simulink model "drone_PID"  (R2021a)
settings: Solver=FixedStepAuto  StartTime=0.0  StopTime=10.0  RelTol=1e-3  EnableMultiTasking=on
model workspace (MAT data in the model file):
  Ts = 0.016
undefined symbols (not defined in the file or in its folder): AUX, dev, DiscIntNeverNeededParam, pwm_output1
libraries: px4Sensorslib x8, px4lib x4, cstblocks x3, simulink x1
settings Model: ExtModeTrigDuration=10  Creator=Kawaguchi  LastModifiedBy=beket
settings SolverCC: PositivePriorityOrder=on
settings OptimizationCC: EnhancedBackFolding=on  PassReuseOutputArgsAs=Individual arguments  ZeroExternalMemoryAtStartup=off  ZeroInternalMemoryAtStartup=off  MaxStackSize=64  OptimizeBlockOrder=speed  DifferentSizesBufferReuse=on  OptimizationCustomize=off  EfficientTunableParamExpr=on
settings DebuggingCC: ParameterTunabilityLossMsg=error
settings HardwareCC: ProdBitPerPointer=32  ProdBitPerSizeT=32  ProdBitPerPtrDiffT=32  ProdLargestAtomicInteger=Long  ProdLargestAtomicFloat=Double  ProdWordSize=32  ProdLongLongMode=on  ProdHWDeviceType=ARM Compatible->ARM Cortex
settings SFSimCC: MATLABDynamicMemAlloc=off  SimTargetLang=C++
settings RTWCC: SystemTargetFile=ert.tlc  HardwareBoard=PX4 Pixhawk 4  TLCOptions="-aInlineSetEventsForThisBaseRateFcn=TLC_FALSE -aSuppressMultiTaskScheduler=TLC_FALSE  -aRateBasedStepFcn=0"  TemplateMakefile=ert_default_tmf  Toolchain=GNU Tools for PX4 Autopilots  TargetLang=C++
settings CodeAppCC: ForceParamTrailComments=on  IgnoreCustomStorageClasses=off  OperatorAnnotations=on  SimulinkDataObjDesc=on  SFDataObjDesc=on  InsertBlockDesc=on
settings ERTTargetCC: ExtModeTransport=3  ExtModeStaticAlloc=on  ExtModeStaticAllocSize=1024  ExtModeMexFile=ext_xcp  ExtModeIntrfLevel=Level2 - Open

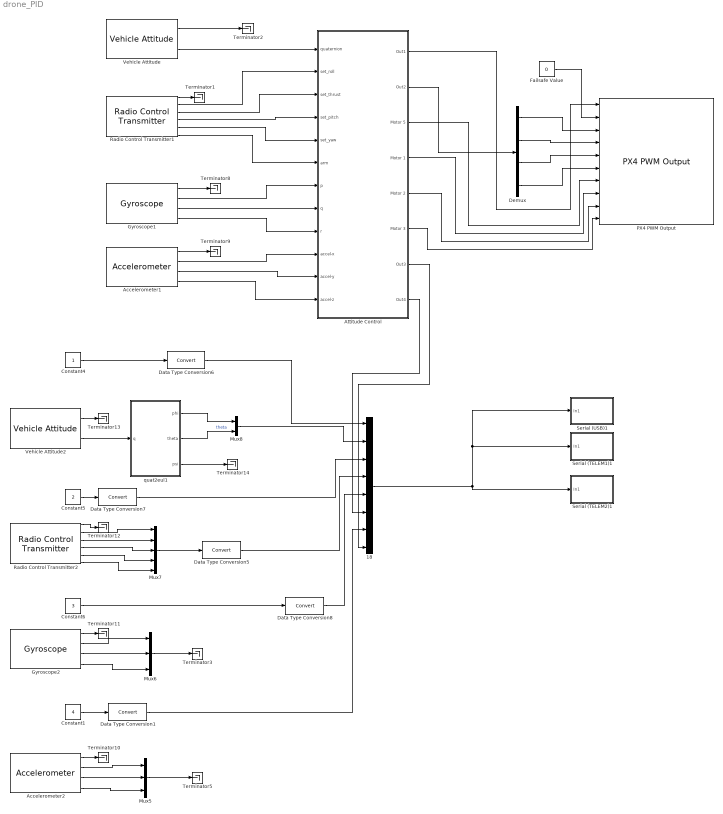
== system drone_PID ==
  18 : Mux  Inputs=8
  Accelerometer1 : px4Sensorslib/Accelerometer  uorbTimeStamp=off  BlockingMode=off  BlockTimeout=1e-3  sampleTime=1/250
      settings: SourceProductBaseCode=PX4AUTOPILOTS
  Accelerometer2 : px4Sensorslib/Accelerometer  uorbTimeStamp=off  BlockingMode=off  BlockTimeout=1e-3  sampleTime=Ts
      settings: SourceProductBaseCode=PX4AUTOPILOTS
  Attitude Control : Subsystem
  Constant1 : Constant  Value=4
  Constant4 : Constant
  Constant5 : Constant  Value=2
  Constant6 : Constant  Value=3
  Data Type Conversion{1,5..8} (5 alike) : DataTypeConversion
  Demux : Demux
  Failsafe Value : Constant  Value=0  OutDataTypeStr=boolean  SampleTime=-1
  Gyroscope1 : px4Sensorslib/Gyroscope  uorbTimeStamp=off  BlockingMode=off  BlockTimeout=1e-3  sampleTime=1/250
      settings: SourceProductBaseCode=PX4AUTOPILOTS
  Gyroscope2 : px4Sensorslib/Gyroscope  uorbTimeStamp=off  BlockingMode=off  BlockTimeout=1e-3  sampleTime=Ts
      settings: SourceProductBaseCode=PX4AUTOPILOTS
  Mux5 : Mux  Inputs=3
  Mux6 : Mux  Inputs=3
  Mux7 : Mux  Inputs=5
  Mux8 : Mux  Inputs=2
  PX4 PWM Output : px4lib/PX4 PWM Output  pwmDevice=AUX (/dev/pwm_output1)  pwmChannel1_=on  pwmChannel2_=on  pwmChannel3_=on  pwmChannel4_=on  pwmChannel5_=on  pwmChannel6_=on  pwmChannel7_=on  pwmChannel8_=on  forceTerminateFailsafe=off  outputErrorStatus=off
      settings: SourceProductBaseCode=PX4AUTOPILOTS
  Radio Control Transmitter1 : px4Sensorslib/Radio Control Transmitter  channel1=on  channel2=on  channel3=on  channel4=on  channel5=on  channel6=off  channel7=off  channel8=off  channel_count=off  rssi=off  rc_input_source=off  timestamp_last_signal=off  time_stamp=off  sampleTime=1/250  BlockingMode=off  BlockTimeout=5
      settings: SourceProductBaseCode=PX4AUTOPILOTS
  Radio Control Transmitter2 : px4Sensorslib/Radio Control Transmitter  channel1=on  channel2=on  channel3=on  channel4=on  channel5=on  channel6=off  channel7=off  channel8=off  channel_count=off  rssi=off  rc_input_source=off  timestamp_last_signal=off  time_stamp=off  sampleTime=Ts  BlockingMode=off  BlockTimeout=5
      settings: SourceProductBaseCode=PX4AUTOPILOTS
  Serial (TELEM1)1 : Subsystem
  Serial (TELEM2)1 : Subsystem
  Serial (USB)1 : Subsystem
  Terminator{1..3,5,8..14} (11 alike) : Terminator
  Vehicle Attitude : px4Sensorslib/Vehicle Attitude  rollRate=off  pitchRate=off  yawRate=off  quaternion=on  uorbTimeStamp=off  BlockingMode=off  BlockTimeout=0.001  sampleTime=1/250
      settings: SourceProductBaseCode=PX4AUTOPILOTS
  Vehicle Attitude2 : px4Sensorslib/Vehicle Attitude  rollRate=off  pitchRate=off  yawRate=off  quaternion=on  uorbTimeStamp=off  BlockingMode=off  BlockTimeout=0.001  sampleTime=Ts
      settings: SourceProductBaseCode=PX4AUTOPILOTS
  quat2eul1 : MATLAB Function  TreatAsAtomicUnit=on
  wires:
  Vehicle Attitude/1 -> Terminator2/1
  Vehicle Attitude/2 -> Attitude Control/1(quaternion)
  Radio Control Transmitter1/1 -> Terminator1/1
  Radio Control Transmitter1/2 -> Attitude Control/2(set_roll)
  Radio Control Transmitter1/3 -> Attitude Control/3(set_thrust)
  Radio Control Transmitter1/4 -> Attitude Control/4(set_pitch)
  Radio Control Transmitter1/5 -> Attitude Control/5(set_yaw)
  Radio Control Transmitter1/6 -> Attitude Control/6(arm)
  Accelerometer1/1 -> Terminator9/1
  Gyroscope1/1 -> Terminator8/1
  Gyroscope1/2 -> Attitude Control/7(p)
  Gyroscope1/3 -> Attitude Control/8(q)
  Gyroscope1/4 -> Attitude Control/9(r)
  Accelerometer1/2 -> Attitude Control/10(accel-x)
  Accelerometer1/3 -> Attitude Control/11(accel-y)
  Accelerometer1/4 -> Attitude Control/12(accel-z)
  Data Type Conversion7/1 -> 18/3
  Accelerometer2/4 -> Mux5/3
  quat2eul1/2(theta) -> Mux8/2  "theta"
  Radio Control Transmitter2/4 -> Mux7/3
  Mux7/1 -> Data Type Conversion5/1
  18/1 -> Serial (TELEM1)1/1(In1), Serial (USB)1/1(In1), Serial (TELEM2)1/1(In1)
  Constant4/1 -> Data Type Conversion6/1
  Constant6/1 -> Data Type Conversion8/1
  Gyroscope2/4 -> Mux6/3
  Data Type Conversion6/1 -> 18/1
  quat2eul1/1(phi) -> Mux8/1
  Radio Control Transmitter2/1 -> Terminator12/1
  Gyroscope2/1 -> Terminator11/1
  Accelerometer2/3 -> Mux5/2
  Constant5/1 -> Data Type Conversion7/1
  Accelerometer2/2 -> Mux5/1
  Data Type Conversion8/1 -> 18/5
  Radio Control Transmitter2/3 -> Mux7/2
  Accelerometer2/1 -> Terminator10/1
  Vehicle Attitude2/1 -> Terminator13/1
  Radio Control Transmitter2/2 -> Mux7/1
  Gyroscope2/3 -> Mux6/2
  quat2eul1/3(psi) -> Terminator14/1
  Gyroscope2/2 -> Mux6/1
  Vehicle Attitude2/2 -> quat2eul1/1(q)
  Mux8/1 -> 18/2
  Data Type Conversion5/1 -> 18/4
  Mux5/1 -> Terminator5/1
  Attitude Control/1(Out1) -> PX4 PWM Output/1
  Demux/1 -> PX4 PWM Output/3
  Demux/2 -> PX4 PWM Output/4
  Demux/3 -> PX4 PWM Output/5
  Demux/4 -> PX4 PWM Output/6
  Failsafe Value/1 -> PX4 PWM Output/2
  Attitude Control/2(Out2) -> Demux/1
  Attitude Control/3(Motor 5) -> PX4 PWM Output/7
  Attitude Control/4(Motor 1) -> PX4 PWM Output/8
  Attitude Control/5(Motor 2) -> PX4 PWM Output/9
  Attitude Control/6(Motor 3) -> PX4 PWM Output/10
  Radio Control Transmitter2/5 -> Mux7/4
  Constant1/1 -> Data Type Conversion1/1
  Attitude Control/7(Out3) -> 18/8
  Data Type Conversion1/1 -> 18/7
  Mux6/1 -> Terminator3/1
  Attitude Control/8(Out4) -> 18/6
  Radio Control Transmitter2/6 -> Mux7/5

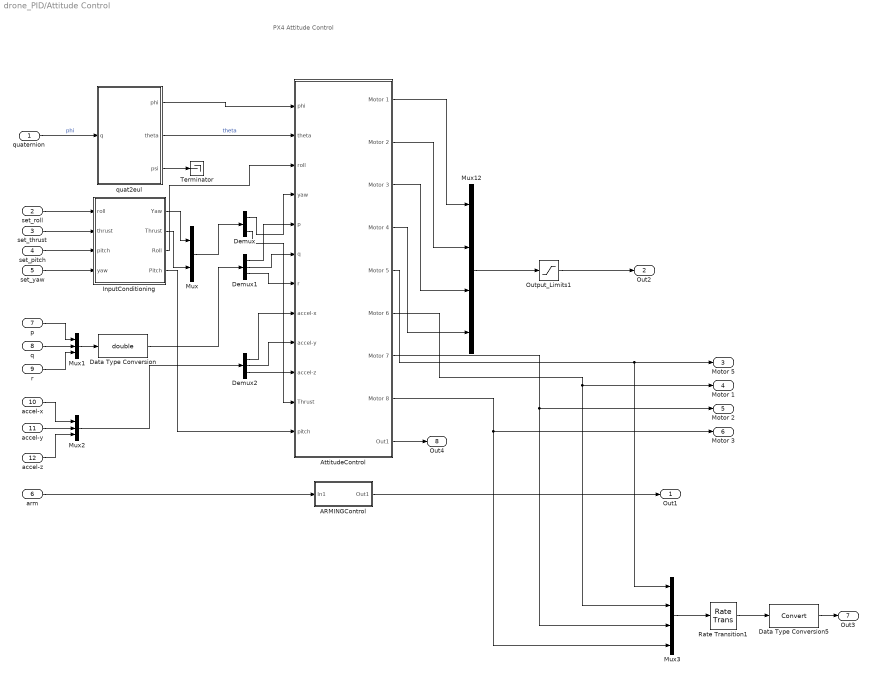
== system drone_PID/Attitude Control ==
  note: PX4 Attitude Control
  quaternion : Inport
  set_roll : Inport  Port=2  OutDataTypeStr=uint16
  set_thrust : Inport  Port=3  OutDataTypeStr=uint16
  set_pitch : Inport  Port=4  OutDataTypeStr=uint16
  set_yaw : Inport  Port=5  OutDataTypeStr=uint16
  arm : Inport  Port=6  OutDataTypeStr=uint16
  p : Inport  Port=7
  q : Inport  Port=8
  r : Inport  Port=9
  accel-x : Inport  Port=10
  accel-y : Inport  Port=11
  accel-z : Inport  Port=12
  ARMINGControl : Subsystem
  AttitudeControl : Subsystem
  Data Type Conversion : DataTypeConversion  OutDataTypeStr=double
  Data Type Conversion5 : DataTypeConversion
  Demux : Demux  Outputs=2
  Demux1 : Demux  Outputs=3
  Demux2 : Demux  Outputs=3
  InputConditioning : Subsystem
  Mux : Mux  Inputs=2
  Mux1 : Mux  Inputs=3
  Mux12 : Mux
  Mux2 : Mux  Inputs=3
  Mux3 : Mux
  Output_Limits1 : Saturate  UpperLimit=2000  LowerLimit=1000
  Rate Transition1 : RateTransition  OutPortSampleTimeOpt=Multiple of input port sample time  OutPortSampleTimeMultiple=4
  Terminator : Terminator
  quat2eul : MATLAB Function  TreatAsAtomicUnit=on
  Out1 : Outport  VectorParamsAs1DForOutWhenUnconnected=off
  Out2 : Outport  Port=2  VectorParamsAs1DForOutWhenUnconnected=off
  Motor 5 : Outport  Port=3  OutDataTypeStr=uint16  VectorParamsAs1DForOutWhenUnconnected=off
  Motor 1 : Outport  Port=4  OutDataTypeStr=uint16  VectorParamsAs1DForOutWhenUnconnected=off
  Motor 2 : Outport  Port=5  OutDataTypeStr=uint16  VectorParamsAs1DForOutWhenUnconnected=off
  Motor 3 : Outport  Port=6  OutDataTypeStr=uint16  VectorParamsAs1DForOutWhenUnconnected=off
  Out3 : Outport  Port=7
  Out4 : Outport  Port=8
  wires:
  set_roll/1 -> InputConditioning/1(roll)
  arm/1 -> ARMINGControl/1(In1)
  quat2eul/2(theta) -> AttitudeControl/2(theta)  "theta"
  Output_Limits1/1 -> Out2/1
  Mux12/1 -> Output_Limits1/1
  ARMINGControl/1(Out1) -> Out1/1
  set_yaw/1 -> InputConditioning/4(yaw)
  quaternion/1 -> quat2eul/1(q)  "phi"
  quat2eul/1(phi) -> AttitudeControl/1(phi)
  quat2eul/3(psi) -> Terminator/1
  AttitudeControl/1(Motor 1) -> Mux12/1
  AttitudeControl/2(Motor 2) -> Mux12/2
  AttitudeControl/3(Motor 3) -> Mux12/3
  AttitudeControl/4(Motor 4) -> Mux12/4
  Mux/1 -> Demux/1
  p/1 -> Mux1/1
  r/1 -> Mux1/3
  Mux1/1 -> Data Type Conversion/1
  Demux1/2 -> AttitudeControl/6(q)
  Demux1/1 -> AttitudeControl/5(p)
  Demux1/3 -> AttitudeControl/7(r)
  accel-y/1 -> Mux2/2
  accel-x/1 -> Mux2/1
  accel-z/1 -> Mux2/3
  Mux2/1 -> Demux2/1
  Demux2/2 -> AttitudeControl/9(accel-y)
  Demux2/1 -> AttitudeControl/8(accel-x)
  Demux2/3 -> AttitudeControl/10(accel-z)
  InputConditioning/1(Yaw) -> Mux/1
  InputConditioning/2(Thrust) -> Mux/2
  Demux/1 -> AttitudeControl/4(yaw)
  Demux/2 -> AttitudeControl/11(Thrust)
  InputConditioning/3(Roll) -> AttitudeControl/3(roll)
  InputConditioning/4(Pitch) -> AttitudeControl/12(pitch)
  set_thrust/1 -> InputConditioning/2(thrust)
  set_pitch/1 -> InputConditioning/3(pitch)
  q/1 -> Mux1/2
  Data Type Conversion/1 -> Demux1/1
  AttitudeControl/5(Motor 5) -> Mux3/1, Motor 5/1
  AttitudeControl/8(Motor 8) -> Mux3/4, Motor 3/1
  AttitudeControl/7(Motor 7) -> Mux3/3, Motor 2/1
  AttitudeControl/6(Motor 6) -> Mux3/2, Motor 1/1
  Mux3/1 -> Rate Transition1/1
  Data Type Conversion5/1 -> Out3/1
  Rate Transition1/1 -> Data Type Conversion5/1
  AttitudeControl/9(Out1) -> Out4/1

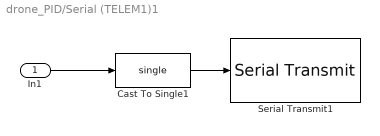
== system drone_PID/Serial (TELEM1)1 ==
  In1 : Inport
  Cast To Single1 : DataTypeConversion  OutDataTypeStr=single
  Serial Transmit1 : px4lib/Serial Transmit  SCIModule=/dev/ttyS1
      settings: SourceProductBaseCode=PX4AUTOPILOTS
  wires:
  Cast To Single1/1 -> Serial Transmit1/1
  In1/1 -> Cast To Single1/1

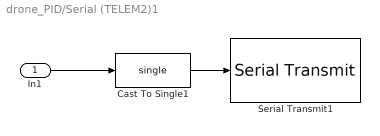
== system drone_PID/Serial (TELEM2)1 ==
  In1 : Inport
  Cast To Single1 : DataTypeConversion  OutDataTypeStr=single
  Serial Transmit1 : px4lib/Serial Transmit  SCIModule=/dev/ttyS2
      settings: SourceProductBaseCode=PX4AUTOPILOTS
  wires:
  Cast To Single1/1 -> Serial Transmit1/1
  In1/1 -> Cast To Single1/1

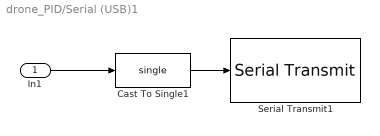
== system drone_PID/Serial (USB)1 ==
  In1 : Inport
  Cast To Single1 : DataTypeConversion  OutDataTypeStr=single
  Serial Transmit1 : px4lib/Serial Transmit  SCIModule=/dev/ttyACM0
      settings: SourceProductBaseCode=PX4AUTOPILOTS
  wires:
  Cast To Single1/1 -> Serial Transmit1/1
  In1/1 -> Cast To Single1/1

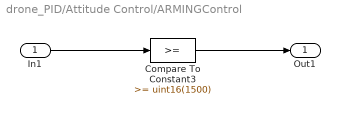
== system drone_PID/Attitude Control/ARMINGControl ==
  In1 : Inport
  Compare To Constant3 : simulink/Logic and Bit Operations/Compare To Constant  relop=>=  const=uint16(1500)  OutDataTypeStr=boolean
  Out1 : Outport  VectorParamsAs1DForOutWhenUnconnected=off
  wires:
  Compare To Constant3/1 -> Out1/1
  In1/1 -> Compare To Constant3/1

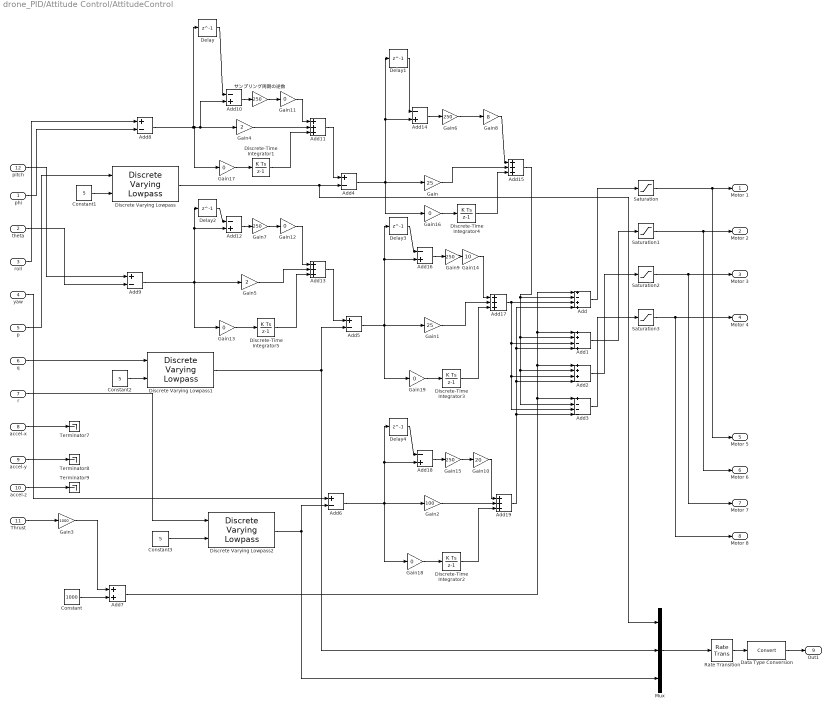
== system drone_PID/Attitude Control/AttitudeControl ==
  phi : Inport
  theta : Inport  Port=2
  roll : Inport  Port=3
  yaw : Inport  Port=4
  p : Inport  Port=5
  q : Inport  Port=6
  r : Inport  Port=7
  accel-x : Inport  Port=8
  accel-y : Inport  Port=9
  accel-z : Inport  Port=10
  Thrust : Inport  Port=11
  pitch : Inport  Port=12
  Add : Sum  Inputs=+-++
  Add1 : Sum  Inputs=++-+
  Add{10,12,14,16,18} (5 alike) : Sum  Inputs=-+
  Add{11,13,15,17,19} (5 alike) : Sum  Inputs=+++
  Add2 : Sum  Inputs=+++-
  Add3 : Sum  Inputs=+---
  Add{4..6,8..9} (5 alike) : Sum  Inputs=+-
  Add7 : Sum
  Constant : Constant  Value=1000
  Constant1 : Constant  Value=5
  Constant2 : Constant  Value=5
  Constant3 : Constant  Value=5
  Data Type Conversion : DataTypeConversion
  Delay{,1..4} (5 alike) : Delay  DelayLength=1  InitialCondition=0
  Discrete Varying Lowpass : cstblocks/Linear Parameter Varying/Discrete Varying Lowpass  N=1  w0=0  Ts=1/250
      settings: SourceProductBaseCode=CT
  Discrete Varying Lowpass1 : cstblocks/Linear Parameter Varying/Discrete Varying Lowpass  N=1  w0=0  Ts=1/250
      settings: SourceProductBaseCode=CT
  Discrete Varying Lowpass2 : cstblocks/Linear Parameter Varying/Discrete Varying Lowpass  N=1  w0=0  Ts=1/250
      settings: SourceProductBaseCode=CT
  Discrete-Time Integrator{1..5} (5 alike) : DiscreteIntegrator  SampleTime=-1  LimitOutput=on  UpperSaturationLimit=5  LowerSaturationLimit=-5  IgnoreLimit=on  ICPrevOutput=DiscIntNeverNeededParam  ICPrevScaledInput=DiscIntNeverNeededParam
  Gain : Gain  Gain=25
  Gain1 : Gain  Gain=25
  Gain10 : Gain  Gain=20
  Gain{11..13,16..19} (7 alike) : Gain  Gain=0
  Gain14 : Gain  Gain=10
  Gain{6..7,9,15} (4 alike) : Gain  Gain=250
  Gain2 : Gain  Gain=100
  Gain3 : Gain  Gain=1000
  Gain4 : Gain  Gain=2
  Gain5 : Gain  Gain=2
  Gain8 : Gain  Gain=8
  Mux : Mux  Inputs=3
  Rate Transition : RateTransition  OutPortSampleTimeOpt=Multiple of input port sample time  OutPortSampleTimeMultiple=4  OutPortSampleTime=4
  Saturation{,1..3} (4 alike) : Saturate  UpperLimit=2000  LowerLimit=800  OutDataTypeStr=uint16
  Terminator7 : Terminator
  Terminator8 : Terminator
  Terminator9 : Terminator
  サンプリング周期の逆数 : Gain  Gain=250
  Motor 1 : Outport  OutDataTypeStr=uint16  VectorParamsAs1DForOutWhenUnconnected=off
  Motor 2 : Outport  Port=2  OutDataTypeStr=uint16  VectorParamsAs1DForOutWhenUnconnected=off
  Motor 3 : Outport  Port=3  OutDataTypeStr=uint16  VectorParamsAs1DForOutWhenUnconnected=off
  Motor 4 : Outport  Port=4  OutDataTypeStr=uint16  VectorParamsAs1DForOutWhenUnconnected=off
  Motor 5 : Outport  Port=5  OutDataTypeStr=uint16  SampleTime=1/250  VectorParamsAs1DForOutWhenUnconnected=off
  Motor 6 : Outport  Port=6  OutDataTypeStr=uint16  VectorParamsAs1DForOutWhenUnconnected=off
  Motor 7 : Outport  Port=7  OutDataTypeStr=uint16  VectorParamsAs1DForOutWhenUnconnected=off
  Motor 8 : Outport  Port=8  OutDataTypeStr=uint16  VectorParamsAs1DForOutWhenUnconnected=off
  Out1 : Outport  Port=9
  wires:
  Add2/1 -> Saturation2/1
  Gain/1 -> Add15/2
  Add17/1 -> Add2/3, Add3/3, Add1/3, Add/3
  Add18/1 -> Gain15/1
  Add13/1 -> Add5/1
  Add14/1 -> Gain6/1
  Gain15/1 -> Gain10/1
  Gain11/1 -> Add11/1
  Gain1/1 -> Add17/2
  Gain3/1 -> Add7/1
  theta/1 -> Add9/2
  Gain14/1 -> Add17/1
  Gain12/1 -> Add13/1
  Gain5/1 -> Add13/2
  Saturation/1 -> Motor 5/1, Motor 1/1
  r/1 -> Discrete Varying Lowpass2/1
  Gain9/1 -> Gain14/1
  Gain6/1 -> Gain8/1
  Gain7/1 -> Gain12/1
  Add19/1 -> Add2/4, Add1/4, Add/4, Add3/4
  Add15/1 -> Add/2, Add1/2, Add2/2, Add3/2
  Add16/1 -> Gain9/1
  accel-z/1 -> Terminator9/1
  Delay3/1 -> Add16/1
  Constant/1 -> Add7/2
  Gain10/1 -> Add19/1
  Delay/1 -> Add10/1
  Gain4/1 -> Add11/2
  サンプリング周期の逆数/1 -> Gain11/1
  Thrust/1 -> Gain3/1
  Delay4/1 -> Add18/1
  Delay2/1 -> Add12/1
  Add11/1 -> Add4/1
  Add12/1 -> Gain7/1
  accel-x/1 -> Terminator7/1
  Add3/1 -> Saturation3/1
  Gain2/1 -> Add19/2
  Saturation2/1 -> Motor 7/1, Motor 3/1
  Add/1 -> Saturation/1
  Add10/1 -> サンプリング周期の逆数/1
  roll/1 -> Add8/1
  phi/1 -> Add8/2
  pitch/1 -> Add9/1
  Saturation3/1 -> Motor 8/1, Motor 4/1
  Add1/1 -> Saturation1/1
  Add7/1 -> Add/1, Add1/1, Add2/1, Add3/1
  accel-y/1 -> Terminator8/1
  Saturation1/1 -> Motor 6/1, Motor 2/1
  p/1 -> Discrete Varying Lowpass/1
  q/1 -> Discrete Varying Lowpass1/1
  Gain8/1 -> Add15/1
  yaw/1 -> Add6/1
  Delay1/1 -> Add14/1
  Gain17/1 -> Discrete-Time Integrator1/1
  Add8/1 -> Gain4/1, Add10/2, Gain17/1, Delay/1
  Discrete-Time Integrator1/1 -> Add11/3
  Gain13/1 -> Discrete-Time Integrator5/1
  Discrete-Time Integrator5/1 -> Add13/3
  Add9/1 -> Gain13/1, Delay2/1, Add12/2, Gain5/1
  Gain16/1 -> Discrete-Time Integrator4/1
  Discrete-Time Integrator4/1 -> Add15/3
  Add4/1 -> Gain16/1, Add14/2, Delay1/1, Gain/1
  Gain19/1 -> Discrete-Time Integrator3/1
  Discrete-Time Integrator3/1 -> Add17/3
  Add5/1 -> Gain19/1, Delay3/1, Add16/2, Gain1/1
  Gain18/1 -> Discrete-Time Integrator2/1
  Discrete-Time Integrator2/1 -> Add19/3
  Add6/1 -> Gain18/1, Delay4/1, Add18/2, Gain2/1
  Discrete Varying Lowpass/1 -> Mux/1, Add4/2
  Constant1/1 -> Discrete Varying Lowpass/2
  Discrete Varying Lowpass1/1 -> Mux/2, Add5/2
  Constant2/1 -> Discrete Varying Lowpass1/2
  Constant3/1 -> Discrete Varying Lowpass2/2
  Discrete Varying Lowpass2/1 -> Mux/3, Add6/2
  Mux/1 -> Rate Transition/1
  Rate Transition/1 -> Data Type Conversion/1
  Data Type Conversion/1 -> Out1/1

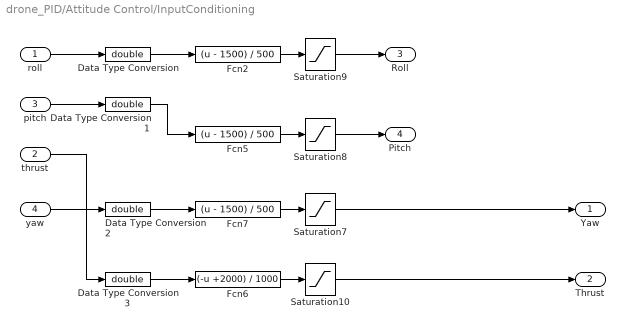
== system drone_PID/Attitude Control/InputConditioning ==
  roll : Inport
  thrust : Inport  Port=2
  pitch : Inport  Port=3
  yaw : Inport  Port=4
  Data Type Conversion{,1..3} (4 alike) : DataTypeConversion  OutDataTypeStr=double
  Fcn2 : Fcn  Expr=(u - 1500) / 500
  Fcn5 : Fcn  Expr=(u - 1500) / 500
  Fcn6 : Fcn  Expr=(-u +2000) / 1000
  Fcn7 : Fcn  Expr=(u - 1500) / 500
  Saturation10 : Saturate  UpperLimit=1  LowerLimit=0
  Saturation7 : Saturate  UpperLimit=1  LowerLimit=-1
  Saturation8 : Saturate  UpperLimit=1  LowerLimit=-1
  Saturation9 : Saturate  UpperLimit=1  LowerLimit=-1
  Yaw : Outport  VectorParamsAs1DForOutWhenUnconnected=off
  Thrust : Outport  Port=2  VectorParamsAs1DForOutWhenUnconnected=off
  Roll : Outport  Port=3  VectorParamsAs1DForOutWhenUnconnected=off
  Pitch : Outport  Port=4  VectorParamsAs1DForOutWhenUnconnected=off
  wires:
  Saturation10/1 -> Thrust/1
  Saturation7/1 -> Yaw/1
  Saturation8/1 -> Pitch/1
  Fcn6/1 -> Saturation10/1
  thrust/1 -> Data Type Conversion3/1
  Fcn2/1 -> Saturation9/1
  Fcn5/1 -> Saturation8/1
  Saturation9/1 -> Roll/1
  Fcn7/1 -> Saturation7/1
  yaw/1 -> Data Type Conversion2/1
  pitch/1 -> Data Type Conversion1/1
  roll/1 -> Data Type Conversion/1
  Data Type Conversion/1 -> Fcn2/1
  Data Type Conversion1/1 -> Fcn5/1
  Data Type Conversion2/1 -> Fcn7/1
  Data Type Conversion3/1 -> Fcn6/1

== matlab function drone_PID/Attitude Control/quat2eul ==
  data: q input; phi output; theta output; psi output
function [phi,theta,psi] = quat2eul(q)

% Quaternion conversion to Euler angles based on the PX4 Firmware v1.6.5
% release.

phi = atan2(2*(q(1)*q(2) + q(3)* q(4)), q(1)^2 - q(2)^2 - q(3)^2 + q(4)^2);
theta = asin(-2*(q(2)*q(4) - q(1)*q(3)));
psi = atan2(2*(q(2)*q(3) + q(1)* q(4)), q(1)^2 + q(2)^2 - q(3)^2 - q(4)^2);

end

== matlab function drone_PID/quat2eul1 ==
  data: q input; phi output; theta output; psi output
function [phi,theta,psi] = quat2eul(q)

% Quaternion conversion to Euler angles based on the PX4 Firmware v1.6.5
% release.

phi = atan2(2*(q(1)*q(2) + q(3)* q(4)), q(1)^2 - q(2)^2 - q(3)^2 + q(4)^2);
theta = asin(-2*(q(2)*q(4) - q(1)*q(3)));
psi = atan2(2*(q(2)*q(3) + q(1)* q(4)), q(1)^2 + q(2)^2 - q(3)^2 - q(4)^2);

end
